simulink model "SecRwRtStZeroCtrl"  (R2018b)
settings: Solver=FixedStepDiscrete  StartTime=0.0  StopTime=10.0  RelTol=1e-3
undefined symbols (not defined in the file or in its folder): KeSMSuMdMotFinshdTm_Val, KeSMSuMdRetryTm1_Val, KeSMSuModeReqDurgTm_Val
libraries: StCtrlLibBkRecln x1
settings Model: Creator=sn2xws  LastModifiedBy=sn55gm
settings Model: ModifiedHistory=|
  | 2024.5.6
  | 557 First Release
  | 2024.8.14 V3.0.0 bitmask改为变量接口
  | 2025.12.04 V3.1.0mode12防夹后退出
settings DataIOCC: SaveFormat=StructureWithTime
settings OptimizationCC: DefaultParameterBehavior=Inlined  EnhancedBackFolding=on  PassReuseOutputArgsAs=Individual arguments  ZeroExternalMemoryAtStartup=off  ZeroInternalMemoryAtStartup=off  OptimizeBlockOrder=speed  DifferentSizesBufferReuse=on  OptimizationCustomize=off
settings DebuggingCC: ParameterTunabilityLossMsg=error
settings SFSimCC: MATLABDynamicMemAlloc=off
settings RTWCC: SystemTargetFile=autosar.tlc  GenCodeOnly=on  TemplateMakefile=ert_default_tmf  Description=AUTOSAR  GenerateReport=on  IncludeHyperlinkInReport=on  LaunchReport=on  GenerateTraceInfo=on  GenerateTraceReport=on  GenerateTraceReportSl=on  GenerateTraceReportSf=on  GenerateTraceReportEml=on
settings CodeAppCC: ForceParamTrailComments=on  IgnoreCustomStorageClasses=off  OperatorAnnotations=on  SimulinkDataObjDesc=on  SFDataObjDesc=on  InsertBlockDesc=on
settings STFCustomTargetCC: TargetLangStandard=C99 (ISO)  MultiwordLength=256  ParMdlRefBuildCompliant=on  CompOptLevelCompliant=on  IncludeMdlTerminateFcn=off  CombineOutputUpdateFcns=on  SuppressErrorStatus=on  ERTCustomFileBanners=on  SupportNonFinite=off  SupportComplex=off  SupportContinuousTime=off  SupportNonInlinedSFcns=off  RemoveResetFunc=on  MATLABClassNameForMDSCustomization=Simulink.SoftwareTarget.ERTCustomization  AutosarCompliant=on  UseToolchainInfoCompliant=on  LookupTableObjectStructAxisOrder=2,1,3,4,...  LUTObjectStructOrderEvenSpacing=Size,Table,Breakpoints  SystemTargetFile=autosar.tlc
settings ERTTargetCC: TargetLangStandard=C99 (ISO)  ConcurrentExecutionCompliant=off  IncludeMdlTerminateFcn=off  SuppressErrorStatus=on  SupportNonFinite=off  SupportComplex=off  ModelStepFunctionPrototypeControlCompliant=off  CPPClassGenCompliant=off  AutosarCompliant=on  LookupTableObjectStructAxisOrder=2,1,3,4,...  LUTObjectStructOrderEvenSpacing=Size,Table,Breakpoints  InlinedParameterPlacement=NonHierarchical  ERTCustomFileTemplate=example_file_process.tlc  ERTFilePackagingFormat=Compact

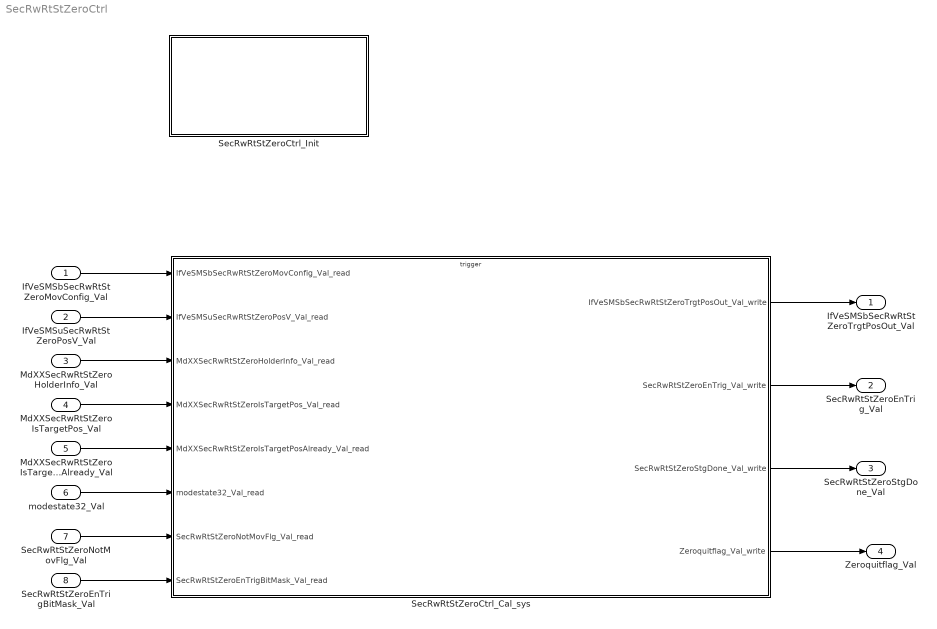
== system SecRwRtStZeroCtrl ==
  IfVeSMSbSecRwRtStZeroMovConfig_Val : Inport  OutDataTypeStr=boolean  PortDimensions=1
  IfVeSMSuSecRwRtStZeroPosV_Val : Inport  Port=2  OutDataTypeStr=boolean  PortDimensions=1
  MdXXSecRwRtStZeroHolderInfo_Val : Inport  Port=3  OutDataTypeStr=uint32  PortDimensions=1
  MdXXSecRwRtStZeroIsTargetPos_Val : Inport  Port=4  OutDataTypeStr=uint32  PortDimensions=1
  MdXXSecRwRtStZeroIsTargetPosAlready_Val : Inport  Port=5  OutDataTypeStr=uint32  PortDimensions=1
  modestate32_Val : Inport  Port=6  OutDataTypeStr=uint32  PortDimensions=1
  SecRwRtStZeroNotMovFlg_Val : Inport  Port=7  OutDataTypeStr=boolean  PortDimensions=1
  SecRwRtStZeroEnTrigBitMask_Val : Inport  Port=8  OutDataTypeStr=uint32  PortDimensions=1
  SecRwRtStZeroCtrl_Cal_sys : Subsystem
  SecRwRtStZeroCtrl_Init : Subsystem
  IfVeSMSbSecRwRtStZeroTrgtPosOut_Val : Outport  OutDataTypeStr=boolean  PortDimensions=1
  SecRwRtStZeroEnTrig_Val : Outport  Port=2  OutDataTypeStr=boolean  PortDimensions=1
  SecRwRtStZeroStgDone_Val : Outport  Port=3  OutDataTypeStr=boolean  PortDimensions=1
  Zeroquitflag_Val : Outport  Port=4  OutDataTypeStr=boolean  PortDimensions=1
  wires:
  IfVeSMSbSecRwRtStZeroMovConfig_Val/1 -> SecRwRtStZeroCtrl_Cal_sys/1(IfVeSMSbSecRwRtStZeroMovConfig_Val_read)
  IfVeSMSuSecRwRtStZeroPosV_Val/1 -> SecRwRtStZeroCtrl_Cal_sys/2(IfVeSMSuSecRwRtStZeroPosV_Val_read)
  MdXXSecRwRtStZeroHolderInfo_Val/1 -> SecRwRtStZeroCtrl_Cal_sys/3(MdXXSecRwRtStZeroHolderInfo_Val_read)
  MdXXSecRwRtStZeroIsTargetPos_Val/1 -> SecRwRtStZeroCtrl_Cal_sys/4(MdXXSecRwRtStZeroIsTargetPos_Val_read)
  MdXXSecRwRtStZeroIsTargetPosAlready_Val/1 -> SecRwRtStZeroCtrl_Cal_sys/5(MdXXSecRwRtStZeroIsTargetPosAlready_Val_read)
  modestate32_Val/1 -> SecRwRtStZeroCtrl_Cal_sys/6(modestate32_Val_read)
  SecRwRtStZeroNotMovFlg_Val/1 -> SecRwRtStZeroCtrl_Cal_sys/7(SecRwRtStZeroNotMovFlg_Val_read)
  SecRwRtStZeroCtrl_Cal_sys/1(IfVeSMSbSecRwRtStZeroTrgtPosOut_Val_write) -> IfVeSMSbSecRwRtStZeroTrgtPosOut_Val/1
  SecRwRtStZeroCtrl_Cal_sys/2(SecRwRtStZeroEnTrig_Val_write) -> SecRwRtStZeroEnTrig_Val/1
  SecRwRtStZeroCtrl_Cal_sys/3(SecRwRtStZeroStgDone_Val_write) -> SecRwRtStZeroStgDone_Val/1
  SecRwRtStZeroEnTrigBitMask_Val/1 -> SecRwRtStZeroCtrl_Cal_sys/8(SecRwRtStZeroEnTrigBitMask_Val_read)
  SecRwRtStZeroCtrl_Cal_sys/4(Zeroquitflag_Val_write) -> Zeroquitflag_Val/1

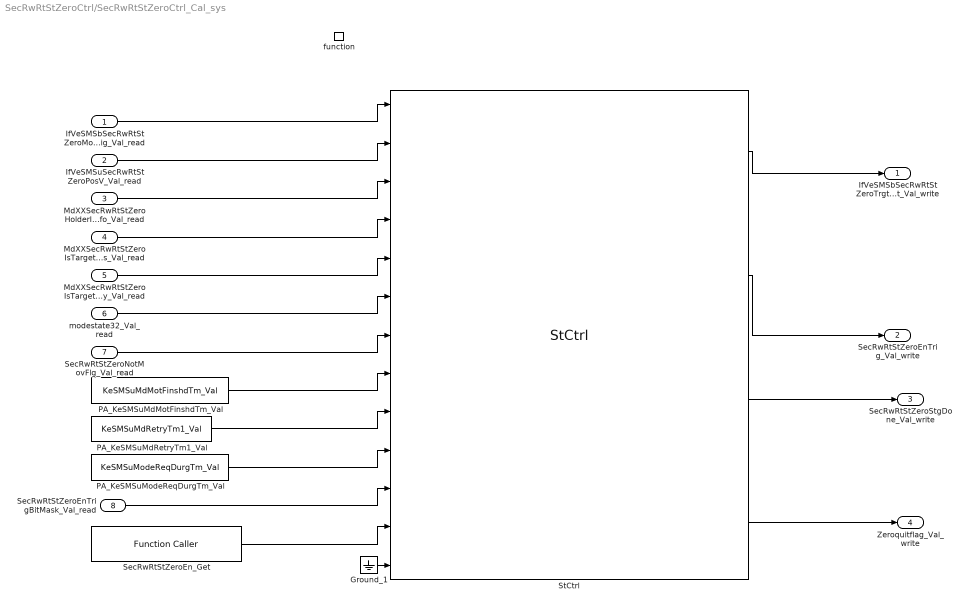
== system SecRwRtStZeroCtrl/SecRwRtStZeroCtrl_Cal_sys ==
  IfVeSMSbSecRwRtStZeroMovConfig_Val_read : Inport
  IfVeSMSuSecRwRtStZeroPosV_Val_read : Inport  Port=2
  MdXXSecRwRtStZeroHolderInfo_Val_read : Inport  Port=3
  MdXXSecRwRtStZeroIsTargetPos_Val_read : Inport  Port=4
  MdXXSecRwRtStZeroIsTargetPosAlready_Val_read : Inport  Port=5
  modestate32_Val_read : Inport  Port=6
  SecRwRtStZeroNotMovFlg_Val_read : Inport  Port=7
  SecRwRtStZeroEnTrigBitMask_Val_read : Inport  Port=8
  function : TriggerPort  TriggerType=function-call  IsSimulinkFunction=on  FunctionName=SecRwRtStZeroCtrl_Cal  VariantControl=(inherit)
  Ground_1 : Ground
  PA_KeSMSuMdMotFinshdTm_Val : Constant  Value=KeSMSuMdMotFinshdTm_Val
  PA_KeSMSuMdRetryTm1_Val : Constant  Value=KeSMSuMdRetryTm1_Val
  PA_KeSMSuModeReqDurgTm_Val : Constant  Value=KeSMSuModeReqDurgTm_Val
  SecRwRtStZeroEn_Get : FunctionCaller  FunctionPrototype=data = SecRwRtStZeroEn_Get()  OutputArgumentSpecifications=uint32(1)
  StCtrl : StCtrlLibBkRecln/StCtrl  SystemSampleTime=-1
  IfVeSMSbSecRwRtStZeroTrgtPosOut_Val_write : Outport
      settings: EnsureOutportIsVirtual=on
  SecRwRtStZeroEnTrig_Val_write : Outport  Port=2
      settings: EnsureOutportIsVirtual=on
  SecRwRtStZeroStgDone_Val_write : Outport  Port=3
      settings: EnsureOutportIsVirtual=on
  Zeroquitflag_Val_write : Outport  Port=4
      settings: EnsureOutportIsVirtual=on
  wires:
  IfVeSMSbSecRwRtStZeroMovConfig_Val_read/1 -> StCtrl/1
  IfVeSMSuSecRwRtStZeroPosV_Val_read/1 -> StCtrl/2
  MdXXSecRwRtStZeroHolderInfo_Val_read/1 -> StCtrl/3
  SecRwRtStZeroNotMovFlg_Val_read/1 -> StCtrl/7
  StCtrl/1 -> IfVeSMSbSecRwRtStZeroTrgtPosOut_Val_write/1
  StCtrl/2 -> SecRwRtStZeroEnTrig_Val_write/1
  StCtrl/3 -> SecRwRtStZeroStgDone_Val_write/1
  SecRwRtStZeroEn_Get/1 -> StCtrl/12
  SecRwRtStZeroEnTrigBitMask_Val_read/1 -> StCtrl/11
  PA_KeSMSuModeReqDurgTm_Val/1 -> StCtrl/10
  PA_KeSMSuMdRetryTm1_Val/1 -> StCtrl/9
  PA_KeSMSuMdMotFinshdTm_Val/1 -> StCtrl/8
  modestate32_Val_read/1 -> StCtrl/6
  MdXXSecRwRtStZeroIsTargetPosAlready_Val_read/1 -> StCtrl/5
  MdXXSecRwRtStZeroIsTargetPos_Val_read/1 -> StCtrl/4
  Ground_1/1 -> StCtrl/13
  StCtrl/4 -> Zeroquitflag_Val_write/1

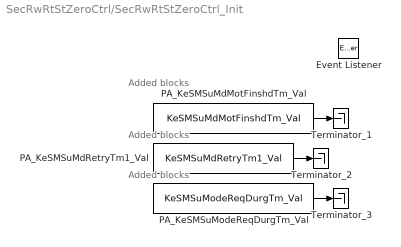
== system SecRwRtStZeroCtrl/SecRwRtStZeroCtrl_Init ==
  note: Added blocks
  note: Added blocks
  note: Added blocks
  Event Listener : EventListener  EventName=reset
  PA_KeSMSuMdMotFinshdTm_Val : Constant  Value=KeSMSuMdMotFinshdTm_Val
  PA_KeSMSuMdRetryTm1_Val : Constant  Value=KeSMSuMdRetryTm1_Val
  PA_KeSMSuModeReqDurgTm_Val : Constant  Value=KeSMSuModeReqDurgTm_Val
  Terminator_1 : Terminator
  Terminator_2 : Terminator
  Terminator_3 : Terminator
  wires:
  PA_KeSMSuMdMotFinshdTm_Val/1 -> Terminator_1/1
  PA_KeSMSuMdRetryTm1_Val/1 -> Terminator_2/1
  PA_KeSMSuModeReqDurgTm_Val/1 -> Terminator_3/1
